simulink model "models"  (R2021a)
settings: Solver=FixedStepAuto  StartTime=0.0  StopTime=10.0  FixedStep=1e-4  RelTol=1e-3
settings Model: Creator=rubro  LastModifiedBy=rubro

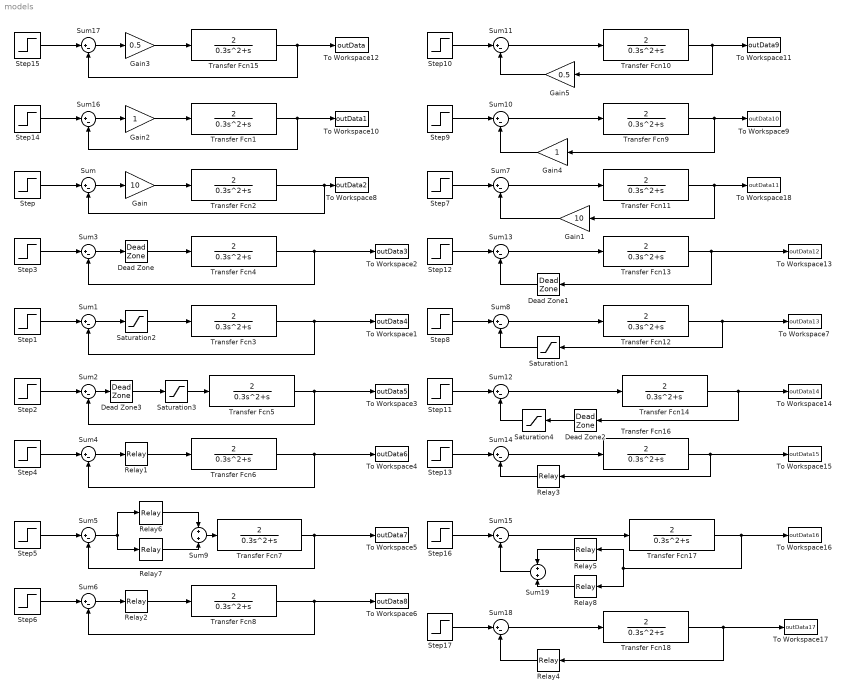
== system models ==
  Dead Zone : DeadZone  LowerValue=-0.1  UpperValue=0.1  SaturateOnIntegerOverflow=on
  Dead Zone1 : DeadZone  LowerValue=-0.1  UpperValue=0.1  SaturateOnIntegerOverflow=on
  Dead Zone2 : DeadZone  LowerValue=-0.4  UpperValue=0.4  SaturateOnIntegerOverflow=on
  Dead Zone3 : DeadZone  LowerValue=-0.4  UpperValue=0.4  SaturateOnIntegerOverflow=on
  Gain : Gain  Gain=10
  Gain1 : Gain  Gain=10
  Gain2 : Gain
  Gain3 : Gain  Gain=0.5
  Gain4 : Gain
  Gain5 : Gain  Gain=0.5
  Relay1 : Relay  OnSwitchValue=0  OffSwitchValue=0  OnOutputValue=0.4  OffOutputValue=-0.4
  Relay2 : Relay  OnSwitchValue=0.1  OffSwitchValue=-0.1  OffOutputValue=-1
  Relay3 : Relay  OnSwitchValue=0  OffSwitchValue=0  OnOutputValue=0.4  OffOutputValue=-0.4
  Relay4 : Relay  OnSwitchValue=0.1  OffSwitchValue=-0.1  OffOutputValue=-1
  Relay5 : Relay  OnSwitchValue=-0.1  OffSwitchValue=-0.1  OnOutputValue=0  OffOutputValue=-1
  Relay6 : Relay  OnSwitchValue=-0.1  OffSwitchValue=-0.1  OnOutputValue=0  OffOutputValue=-1
  Relay7 : Relay  OnSwitchValue=0.1  OffSwitchValue=0.1
  Relay8 : Relay  OnSwitchValue=0.1  OffSwitchValue=0.1
  Saturation{1..4} (4 alike) : Saturate  UpperLimit=1  LowerLimit=-1
  Step{,1..17} (18 alike) : Step  Time=0  SampleTime=0
  Sum{,1..8,10..18} (18 alike) : Sum  Inputs=|+-
  Sum19 : Sum
  Sum9 : Sum
  To Workspace1 : ToWorkspace  VariableName=outData4  SampleTime=-1
  To Workspace10 : ToWorkspace  VariableName=outData1  SampleTime=-1
  To Workspace11 : ToWorkspace  VariableName=outData9  SampleTime=-1
  To Workspace12 : ToWorkspace  VariableName=outData  SampleTime=-1
  To Workspace13 : ToWorkspace  VariableName=outData12  SampleTime=-1
  To Workspace14 : ToWorkspace  VariableName=outData14  SampleTime=-1
  To Workspace15 : ToWorkspace  VariableName=outData15  SampleTime=-1
  To Workspace16 : ToWorkspace  VariableName=outData16  SampleTime=-1
  To Workspace17 : ToWorkspace  VariableName=outData17  SampleTime=-1
  To Workspace18 : ToWorkspace  VariableName=outData11  SampleTime=-1
  To Workspace2 : ToWorkspace  VariableName=outData3  SampleTime=-1
  To Workspace3 : ToWorkspace  VariableName=outData5  SampleTime=-1
  To Workspace4 : ToWorkspace  VariableName=outData6  SampleTime=-1
  To Workspace5 : ToWorkspace  VariableName=outData7  SampleTime=-1
  To Workspace6 : ToWorkspace  VariableName=outData8  SampleTime=-1
  To Workspace7 : ToWorkspace  VariableName=outData13  SampleTime=-1
  To Workspace8 : ToWorkspace  VariableName=outData2  SampleTime=-1
  To Workspace9 : ToWorkspace  VariableName=outData10  SampleTime=-1
  Transfer Fcn{1..18} (18 alike) : TransferFcn  Numerator=[2]  Denominator=[0.3 1 0]
  wires:
  Sum16/1 -> Gain2/1
  Step14/1 -> Sum16/1
  Transfer Fcn1/1 -> Sum16/2, To Workspace10/1
  Sum17/1 -> Gain3/1
  Transfer Fcn15/1 -> To Workspace12/1, Sum17/2
  Gain3/1 -> Transfer Fcn15/1
  Step15/1 -> Sum17/1
  Gain2/1 -> Transfer Fcn1/1
  Transfer Fcn2/1 -> To Workspace8/1, Sum/2
  Gain/1 -> Transfer Fcn2/1
  Step/1 -> Sum/1
  Sum/1 -> Gain/1
  Sum3/1 -> Dead Zone/1
  Step3/1 -> Sum3/1
  Dead Zone/1 -> Transfer Fcn4/1
  Transfer Fcn4/1 -> Sum3/2, To Workspace2/1
  Sum1/1 -> Saturation2/1
  Saturation2/1 -> Transfer Fcn3/1
  Transfer Fcn3/1 -> Sum1/2, To Workspace1/1
  Step1/1 -> Sum1/1
  Step2/1 -> Sum2/1
  Transfer Fcn5/1 -> Sum2/2, To Workspace3/1
  Dead Zone3/1 -> Saturation3/1
  Sum2/1 -> Dead Zone3/1
  Saturation3/1 -> Transfer Fcn5/1
  Relay1/1 -> Transfer Fcn6/1
  Step4/1 -> Sum4/1
  Transfer Fcn6/1 -> Sum4/2, To Workspace4/1
  Sum4/1 -> Relay1/1
  Relay7/1 -> Sum9/2
  Sum5/1 -> Relay6/1, Relay7/1
  Relay6/1 -> Sum9/1
  Transfer Fcn7/1 -> Sum5/2, To Workspace5/1
  Step5/1 -> Sum5/1
  Sum9/1 -> Transfer Fcn7/1
  Sum6/1 -> Relay2/1
  Transfer Fcn8/1 -> To Workspace6/1, Sum6/2
  Step6/1 -> Sum6/1
  Relay2/1 -> Transfer Fcn8/1
  Step17/1 -> Sum18/1
  Transfer Fcn18/1 -> Relay4/1, To Workspace17/1
  Step16/1 -> Sum15/1
  Relay5/1 -> Sum19/1
  Relay8/1 -> Sum19/2
  Transfer Fcn16/1 -> Relay3/1, To Workspace15/1
  Step13/1 -> Sum14/1
  Transfer Fcn14/1 -> Dead Zone2/1, To Workspace14/1
  Step11/1 -> Sum12/1
  Step8/1 -> Sum8/1
  Transfer Fcn12/1 -> Saturation1/1, To Workspace7/1
  Transfer Fcn13/1 -> Dead Zone1/1, To Workspace13/1
  Step12/1 -> Sum13/1
  Step7/1 -> Sum7/1
  Transfer Fcn11/1 -> Gain1/1, To Workspace18/1
  Step10/1 -> Sum11/1
  Transfer Fcn10/1 -> Gain5/1, To Workspace11/1
  Transfer Fcn9/1 -> Gain4/1, To Workspace9/1
  Step9/1 -> Sum10/1
  Sum7/1 -> Transfer Fcn11/1
  Gain1/1 -> Sum7/2
  Sum10/1 -> Transfer Fcn9/1
  Gain4/1 -> Sum10/2
  Gain5/1 -> Sum11/2
  Sum11/1 -> Transfer Fcn10/1
  Sum13/1 -> Transfer Fcn13/1
  Dead Zone1/1 -> Sum13/2
  Sum8/1 -> Transfer Fcn12/1
  Saturation1/1 -> Sum8/2
  Sum12/1 -> Transfer Fcn14/1
  Dead Zone2/1 -> Saturation4/1
  Saturation4/1 -> Sum12/2
  Relay3/1 -> Sum14/2
  Sum14/1 -> Transfer Fcn16/1
  Sum19/1 -> Sum15/2
  Sum15/1 -> Transfer Fcn17/1
  Transfer Fcn17/1 -> Relay5/1, Relay8/1, To Workspace16/1
  Relay4/1 -> Sum18/2
  Sum18/1 -> Transfer Fcn18/1
